simulink model "eas4710_waypoint_block_modified"  (Simulink 10.0)
settings: Solver=ode45  StartTime=0.0  StopTime=30.0  RelTol=1e-3  EnableMultiTasking=on
values from neighbouring files (symbols this model uses):
  Kp = 0.005    [lind_latd_New_Wing.m]
  Kr = 0.85    [lind_latd_New_Wing.m]
  V = [Xdot;Ydot;Zdot]    [eas4710_waypoint_xyz.m]
undefined symbols (not defined in the file or in its folder): Aact, Aele, Alatd, Along, Atau, Bact, Bele, Blatd, Blong, Btau, Cact, Cele, Clatd, Clong, Ctau, Dact, Dele, Dlatd, Dlong, Dtau, Kd, Kh, Khh, Kk, Kq, Kt
settings Model: LogicAnalyzerSignalOrdering=7688e0d8-0073-437d-a6bf-21ac11d6e4c7,278bfc93-647a-46c5-860c-4fed7e601c0a,e8811ab8-2ef3-4609-b7e3-d09a97d21e11,5258265e-ef5c-44c1-9a10-0ecd99780bbe,4c32fc0e-dbbe-43a7-8c32-e800527402bd,4ed74f00-070e-49d6-a2e0-84de2592670a,454e0bcf-c6a8-4520-a6a7-b41a38302bd2,42e2f258-a5ac-459d-91e5-1c940f2b5424,6e12cf6e-ae7d-4147-8469-3a1837520d71,ccef801c-96ba-4674-ad6f-6285bb897aae,f68f9d77-1217-4aa4-a010-6b5fdf804d61,20fb79e8-d082-4ff8-8e32-b8ceccfae481,3a3133f8-bd8f-4a5b-a583-a2cf637debb2,3cc70fcf-8d10-4e0e-8469-d250dfff0f44,261df20c-dffa-4fcf-856f-8cbb40fcad07,f650f37b-5abe-4a1a-b8ed-fe47acfd593c,ddbe1cf6-8d76-49d3-ae1c-cfd5f55c2b3e  Creator=rick  LastModifiedBy=jsoven  EnablePacing=on  PacingRate=0.890000  ExtModeAutoUpdateStatusClock=off
settings Model: SuppressorTable=|
  | <?xml version="1.0" encoding="UTF-8" standalone="yes" ?>
  | <!DOCTYPE boost_serialization>
  | <boost_serialization signature="serialization::archive" version="15">
  | <DiagnosticSuppressor class_id="0" tracking_level="0" version="6">
  | 	<Table class_id="1" tracking_level="0" version="0">
  | 		<count>2</count>
  | 		<bucket_count>8</bucket_count>
  | 		<item_version>0</item_version>
  | 		<item class_id="2" tracking_level="0" version="0">
  | 			<first class_id="3" tracking_level="0" version="6">
  | 				<Source class_id="4" tracking_level="0" version="0">
  | 					<count>1</count>
  | 					<item_version>0</item_version>
  | 					<item>eas4710_waypoint_block_modified/Product1</item>
  | 				</Source>
  | 			</first>
  | 			<second class_id="5" tracking_level="0" version="6">
  | 				<SuppressedData class_id="6" tracking_level="0" version="0">
  | 					<count>1</count>
  | 					<bucket_count>8</bucket_count>
  | 					<item_version>0</item_version>
  | 					<item class_id="7" tracking_level="0" version="0">
  | 						<first class_id="8" tracking_level="0" version="6">
  | 							<ID>Simulink:blocks:DivideByZero</ID>
  | 							<Cause>
  | 								<Source>
  | 									<count>0</count>
  | 									<item_version>0</item_version>
  | 								</Source>
  | 							</Cause>
  | 						</first>
  | 						<second class_id="9" tracking_level="0" version="6">
  | 							<Comment></Comment>
  | 							<User>jsoven</User>
  | 							<LastModified class_id="10" tracking_level="0" version="0">
  | 								<ptime_date class_id="11" tracking_level="0" version="0">
  | 									<date>20200319</date>
  | 								</ptime_date>
  | 								<ptime_time_duration class_id="12" tracking_level="0" version="0">
  | 									<is_special>0</is_special>
  | 									<time_duration_hours>22</time_duration_hours>
  | 									<time_duration_minutes>15</time_duration_minutes>
  | 									<time_duration_seconds>21</time_duration_seconds>
  | 									<time_duration_fractional_seconds>0</time_duration_fractional_seconds>
  | 								</ptime_time_duration>
  | 							</LastModified>
  | 							<SuppressionType>0</SuppressionType>
  | 						</second>
  | 					</item>
  | 				</SuppressedData>
  | 			</second>
  | 		</item>
  | 		<item>
  | 			<first>
  | 				<Source>
  | 					<count>1</count>
  | 					<item_version>0</item_version>
  | 					<item>eas4710_waypoint_block_modified/Product</item>
  | 				</Source>
  | 			</first>
  | 			<second>
  | 				<SuppressedData>
  | 					<count>1</count>
  | 					<bucket_count>8</bucket_count>
  | 					<item_version>0</item_version>
  | 					<item>
  | 						<first>
  | 							<ID>Simulink:blocks:DivideByZero</ID>
  | 							<Cause>
  | 								<Source>
  | 									<count>0</count>
  | 									<item_version>0</item_version>
  | 								</Source>
  | 							</Cause>
  | 						</first>
  | 						<second>
  | 							<Comment></Comment>
  | 							<User>jsoven</User>
  | 							<LastModified>
  | 								<ptime_date>
  | 									<date>20200319</date>
  | 								</ptime_date>
  | 								<ptime_time_duration>
  | 									<is_special>0</is_special>
  | 									<time_duration_hours>22</time_duration_hours>
  | 									<time_duration_minutes>15</time_duration_minutes>
  | 									<time_duration_seconds>21</time_duration_seconds>
  | 									<time_duration_fractional_seconds>0</time_duration_fractional_seconds>
  | 								</ptime_time_duration>
  | 							</LastModified>
  | 							<SuppressionType>0</SuppressionType>
  | 						</second>
  | 					</item>
  | 				</SuppressedData>
  | 			</second>
  | 		</item>
  | 	</Table>
  | </DiagnosticSuppressor>
  | </boost_serialization>
settings Model: LogicAnalyzerGraphicalSettings=|
  | {
  |   "cursors" : {
  |     "activeCursor" : 0,
  |     "lockedCursors" : [
  | 
  |     ],
  |     "startingCursor" : 0,
  |     "times" : [
  |       0
  |     ]
  |   },
  |   "global" : {
  |   },
  |   "panels" : [
  |     {
  |       "height" : 100,
  |       "startingTrace" : 0,
  |       "traces" : [
  |         {
  |           "signalId" : "7688e0d8-0073-437d-a6bf-21ac11d6e4c7",
  |           "type" : "wave"
  |         },
  |         {
  |           "signalId" : "278bfc93-647a-46c5-860c-4fed7e601c0a",
  |           "type" : "wave"
  |         },
  |         {
  |           "signalId" : "5258265e-ef5c-44c1-9a10-0ecd99780bbe",
  |           "type" : "wave"
  |         },
  |         {
  |           "signalId" : "4ed74f00-070e-49d6-a2e0-84de2592670a",
  |           "type" : "wave"
  |         },
  |         {
  |           "signalId" : "454e0bcf-c6a8-4520-a6a7-b41a38302bd2",
  |           "type" : "wave"
  |         },
  |         {
  |           "signalId" : "42e2f258-a5ac-459d-91e5-1c940f2b5424",
  |           "type" : "wave"
  |         },
  |         {
  |           "signalId" : "f68f9d77-1217-4aa4-a010-6b5fdf804d61",
  |           "type" : "wave"
  |         },
  |         {
  |           "signalId" : "b98533ae-6919-48b8-8c16-58e3b0922f78",
  |           "type" : "wave"
  |         },
  |         {
  |           "signalId" : "245f892d-fdfb-49ac-9386-4648cc77bb9b",
  |           "type" : "wave"
  |         }
  |       ],
  |       "yOffset" : 0
  |     }
  |   ],
  |   "timeAxis" : {
  |     "pixelsPerSecond" : 29.3
  |   },
  |   "trigger" : {
  |     "enabled" : false,
  |     "mode" : "once",
  |     "samples" : 200,
  |     "signals" : {
  |     },
  |     "stages" : [
  |       {
  |         "conditions" : [
  | 
  |         ],
  |         "operator" : "AND"
  |       }
  |     ]
  |   }
  | }
settings DataIOCC: LimitDataPoints=on
settings OptimizationCC: ExpressionDepthLimit=2147483647  InitFltsAndDblsToZero=on
settings DebuggingCC: SaveWithParameterizedLinksMsg=none  SignalResolutionControl=TryResolveAllWithWarning  MultiTaskDSMMsg=warning  MultiTaskCondExecSysMsg=none  FcnCallInpInsideContextMsg=warning  StateNameClashWarn=warning
settings GRTTargetCC: TargetFcnLib=ansi_tfl_tmw.mat  GeneratePreprocessorConditionals=Disable all
settings ConfigComp: CovExternalEMLEnable=off

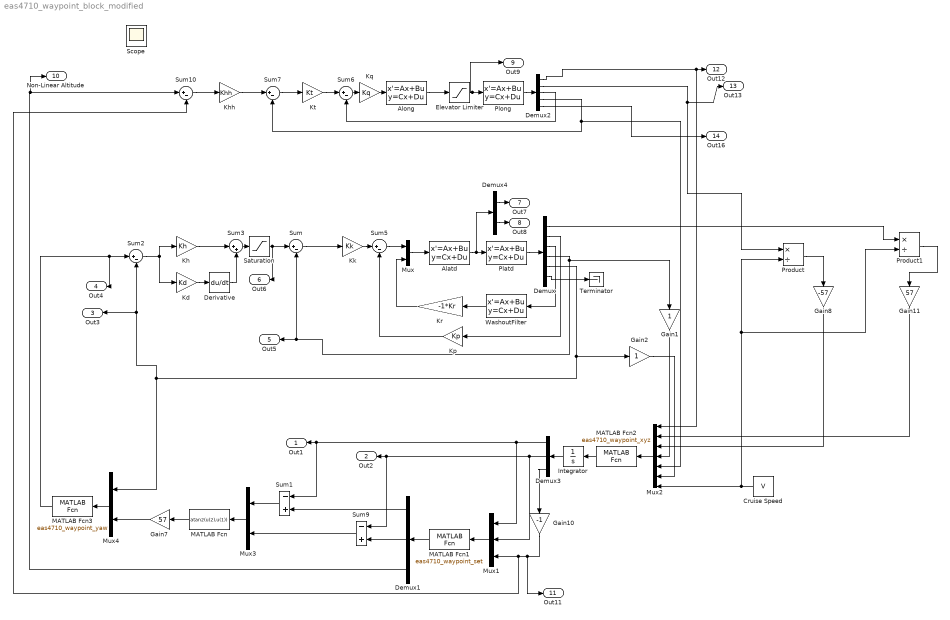
== system eas4710_waypoint_block_modified ==
  Alatd : StateSpace  A=Aact  B=Bact  C=Cact  D=Dact  InitialCondition=0
  Along : StateSpace  A=Aele  B=Bele  C=Cele  D=Dele  InitialCondition=0
  Cruise Speed : Constant  Value=V
  Demux : Demux  Outputs=6
  Demux1 : Demux  Outputs=3
  Demux2 : Demux  Outputs=5
  Demux3 : Demux  Outputs=3
  Demux4 : Demux  Outputs=2
  Derivative : Derivative
  Elevator Limiter : Saturate  UpperLimit=.9  LowerLimit=-.9
  Gain1 : Gain
  Gain10 : Gain  Gain=-1
  Gain11 : Gain  Gain=57
  Gain2 : Gain
  Gain7 : Gain  Gain=57
  Gain8 : Gain  Gain=-57
  Integrator : Integrator
  Kd : Gain  Gain=Kd
  Kh : Gain  Gain=Kh
  Khh : Gain  Gain=Khh
  Kk : Gain  Gain=Kk
  Kp : Gain  Gain=Kp
  Kq : Gain  Gain=Kq
  Kr : Gain  Gain=-1*Kr
  Kt : Gain  Description=Kt  Gain=Kt
  MATLAB Fcn : MATLABFcn  MATLABFcn=atan2(u(2),u(1))
  MATLAB Fcn1 : MATLABFcn  MATLABFcn=eas4710_waypoint_set
  MATLAB Fcn2 : MATLABFcn  MATLABFcn=eas4710_waypoint_xyz
  MATLAB Fcn3 : MATLABFcn  MATLABFcn=eas4710_waypoint_yaw  OutputDimensions=1
  Mux : Mux  Inputs=2
  Mux1 : Mux  Inputs=3
  Mux2 : Mux  Inputs=7
  Mux3 : Mux  Inputs=2
  Mux4 : Mux  Inputs=2
  Platd : StateSpace  A=Alatd  B=Blatd  C=Clatd  D=Dlatd  InitialCondition=0
  Plong : StateSpace  A=Along  B=Blong  C=Clong  D=Dlong  InitialCondition=0
  Product : Product  Inputs=*/
  Product1 : Product  Inputs=*/
  Saturation : Saturate  UpperLimit=45  LowerLimit=-45
  Sum{,2,5..7,10} (6 alike) : Sum  Inputs=|+-
  Sum1 : Sum  Inputs=-+
  Sum3 : Sum  Inputs=|++
  Sum9 : Sum  Inputs=-+
  Terminator : Terminator
  WashoutFilter : StateSpace  A=Atau  B=Btau  C=Ctau  D=Dtau  InitialCondition=0
  Out1 : Outport
  Out2 : Outport  Port=2
  Out3 : Outport  Port=3
  Out4 : Outport  Port=4
  Out5 : Outport  Port=5
  Out6 : Outport  Port=6
  Out7 : Outport  Port=7
  Out8 : Outport  Port=8
  Out9 : Outport  Port=9
  Non-Linear Altitude : Outport  Port=10
  Out11 : Outport  Port=11
  Out12 : Outport  Port=12
  Out13 : Outport  Port=13
  Out16 : Outport  Port=14
  Scope : Scope
  wires:
  Alatd/1 -> Platd/1, Demux4/1
  Platd/1 -> Demux/1
  Mux/1 -> Alatd/1
  Sum5/1 -> Mux/1
  Kh/1 -> Sum3/1
  Sum3/1 -> Saturation/1
  Sum2/1 -> Kh/1, Kd/1
  Derivative/1 -> Sum3/2
  Kd/1 -> Derivative/1
  WashoutFilter/1 -> Kr/1
  Sum9/1 -> Mux3/2
  Sum1/1 -> Mux3/1
  MATLAB Fcn1/1 -> Demux1/1
  Mux1/1 -> MATLAB Fcn1/1
  Along/1 -> Elevator Limiter/1
  Plong/1 -> Demux2/1
  Kt/1 -> Sum6/1
  Sum7/1 -> Kt/1
  Demux1/3 -> Sum10/1, Non-Linear Altitude/1
  MATLAB Fcn2/1 -> Integrator/1
  Integrator/1 -> Demux3/1
  Mux2/1 -> MATLAB Fcn2/1
  Demux3/1 -> Mux1/1, Sum1/1, Out1/1
  Demux3/2 -> Mux1/2, Sum9/1, Out2/1
  Mux3/1 -> MATLAB Fcn/1
  Demux4/1 -> Out7/1
  Demux4/2 -> Out8/1
  MATLAB Fcn/1 -> Gain7/1
  Gain7/1 -> Mux4/2
  Mux4/1 -> MATLAB Fcn3/1
  Demux2/1 -> Mux2/1, Out12/1
  Demux1/2 -> Sum9/2
  Demux1/1 -> Sum1/2
  Sum6/1 -> Kq/1
  Khh/1 -> Sum7/1
  Sum10/1 -> Khh/1
  Demux3/3 -> Gain10/1
  Kr/1 -> Mux/2
  Demux/4 -> Gain1/1, Sum/2, Out5/1
  Kp/1 -> Sum5/2
  Kk/1 -> Sum5/1
  Saturation/1 -> Sum/1, Out6/1
  Demux2/3 -> Sum6/2
  Demux2/4 -> Mux2/5, Sum7/2
  Demux2/5 -> Out16/1
  Demux2/2 -> Product/1, Out13/1
  Cruise Speed/1 -> Product1/2, Product/2, Mux2/7
  Product/1 -> Gain8/1
  Gain8/1 -> Mux2/3
  Gain10/1 -> Sum10/2, Mux1/3, Out11/1
  Demux/1 -> Product1/1
  Product1/1 -> Gain11/1
  Gain11/1 -> Mux2/2
  Demux/3 -> WashoutFilter/1
  Demux/2 -> Kp/1
  Demux/6 -> Terminator/1
  Kq/1 -> Along/1
  Elevator Limiter/1 -> Out9/1, Plong/1
  Gain1/1 -> Mux2/4
  Gain2/1 -> Mux2/6
  Demux/5 -> Gain2/1, Out3/1, Sum2/2, Mux4/1
  Sum/1 -> Kk/1
  MATLAB Fcn3/1 -> Out4/1, Sum2/1
